simulink model "a11_smlk"  (R2023b)
settings: Solver=ode45  StartTime=0.0  StopTime=3  RelTol=1e-3  EnableMultiTasking=on
values from neighbouring files (symbols this model uses):
  A = [-a-b  0  0 ... (first row only)    [a10_obs_contrls.m]    (also in a11_.m = [ 0   1; a12_.m = [ 0   1; a8_conversao_de_formas.m = [ 0  1; a8_state_space.m = [  0      1)
  alpha = inv((C-D*K)*inv(B*K-A)*B+D)    [a11_.m]    (also in a12_.m; a6_.m = 136.626132179)
  B = [ 1 ... (first row only)    [a10_obs_contrls.m]    (also in a11_.m = [ 0; a12_.m = [ 0; a8_conversao_de_formas.m = [ 0; a8_state_space.m = [ 0)
  C = [0 0 1]    [a10_obs_contrls.m]    (also in a11_.m = [ 1 0 ]; a12_.m = [ 1 0 ]; a3_exercicio.m = (s+2)/(s+1); a8_conversao_de_formas.m = [ 5  3 ])
  D = 0    [a11_.m]    (also in a12_.m; a5_sintonia.m = 1.2; a8_conversao_de_formas.m = 1; a8_state_space.m = [ 0 ])
  K = [ 102 19 ]    [a11_.m]    (also in a12_.m; a3_exercicio.m = 0.0938642036672; a4_exercicio.m = 0.2455; a5_sintonia.m = 23.8830609513)
  r = 45    [a11_.m]    (also in a12_.m)
  x0 = [ 30 ... (first row only)    [a11_.m]    (also in a12_.m; a8_state_space.m = [ 1)
settings Model: Creator=andre.bergmann  LastModifiedBy=LUCAS
settings SolverCC: AlgebraicLoopSolver=TrustRegion
settings DataIOCC: LimitDataPoints=on  SaveFormat=Array  ReturnWorkspaceOutputs=off
settings OptimizationCC: ExpressionDepthLimit=2147483647  LifeSpan=inf
settings DebuggingCC: UnderspecifiedInitializationDetection=Classic  MergeDetectMultiDrivingBlocksExec=none  SolverPrmCheckMsg=warning  UnconnectedInputMsg=warning  UnconnectedOutputMsg=warning  UnconnectedLineMsg=warning  StateNameClashWarn=warning  SFUnexpectedBacktrackingDiag=warning  SFNoUnconditionalDefaultTransitionDiag=warning  SFExecutionAtInitializationDiag=none  ArithmeticOperatorsInVariantConditions=warning
settings HardwareCC: ProdBitPerPointer=32  ProdBitPerSizeT=32  ProdBitPerPtrDiffT=32  ProdLargestAtomicFloat=None  ProdIntDivRoundTo=Undefined  ProdEndianess=Unspecified  ProdWordSize=32  ProdHWDeviceType=32-bit Generic
settings ModelReferenceCC: PropagateSignalLabelsOutOfModel=off
settings SFSimCC: SimUseLocalCustomCode=off  CustomCodeUndefinedFunction=UseInterfaceOnly
settings RTWCC: RTWUseLocalCustomCode=off
settings CodeAppCC: StateflowObjectComments=on
settings GRTTargetCC: TargetLangStandard=C89/C90 (ANSI)
settings ConfigComp: CovMetricSettings=dw  CovSaveCumulativeToWorkspaceVar=on  CovSaveSingleToWorkspaceVar=on  CovExternalEMLEnable=off

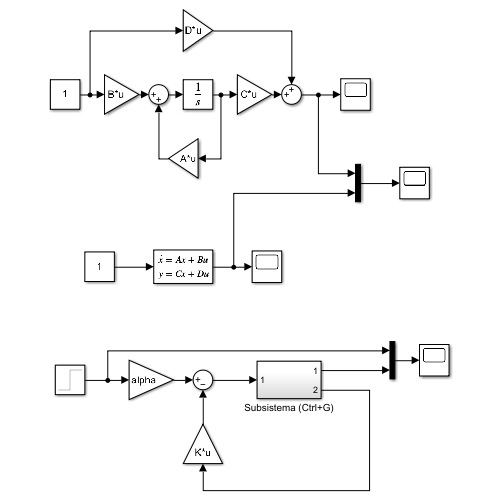
[thumbnail: Simulink's stored preview of the top-level diagram]
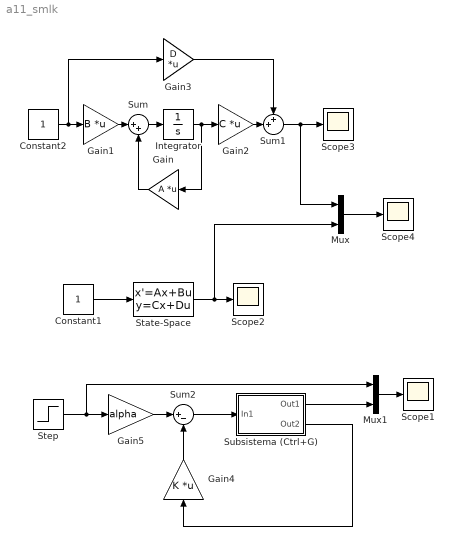
== system a11_smlk ==
  Constant1 : Constant
  Constant2 : Constant
  Gain : Gain  Gain=A  Multiplication=Matrix(K*u)
  Gain1 : Gain  Gain=B  Multiplication=Matrix(K*u)
  Gain2 : Gain  Gain=C  Multiplication=Matrix(K*u)
  Gain3 : Gain  Gain=D  Multiplication=Matrix(K*u)
  Gain4 : Gain  Gain=K  Multiplication=Matrix(K*u)
  Gain5 : Gain  Gain=alpha
  Integrator : Integrator  InitialCondition=x0
  Mux : Mux  Inputs=2
  Mux1 : Mux  Inputs=2
  Scope{1..4} (4 alike) : Scope
  State-Space : StateSpace  A=A  B=B  C=C  D=D  InitialCondition=x0
  Step : Step  After=r  SampleTime=0
  Subsistema (Ctrl+G) : Subsystem
  Sum : Sum  Inputs=|++
  Sum1 : Sum  Inputs=++|
  Sum2 : Sum  Inputs=|+-
  wires:
  Sum2/1 -> Subsistema (Ctrl+G)/1(In1)
  Subsistema (Ctrl+G)/1(Out1) -> Mux1/2
  Subsistema (Ctrl+G)/2(Out2) -> Gain4/1
  Constant1/1 -> State-Space/1
  State-Space/1 -> Mux/2, Scope2/1
  Constant2/1 -> Gain3/1, Gain1/1
  Gain/1 -> Sum/2
  Sum/1 -> Integrator/1
  Sum1/1 -> Mux/1, Scope3/1
  Gain2/1 -> Sum1/2
  Integrator/1 -> Gain2/1, Gain/1
  Gain3/1 -> Sum1/1
  Gain1/1 -> Sum/1
  Mux/1 -> Scope4/1
  Mux1/1 -> Scope1/1
  Gain4/1 -> Sum2/2
  Step/1 -> Mux1/1, Gain5/1
  Gain5/1 -> Sum2/1

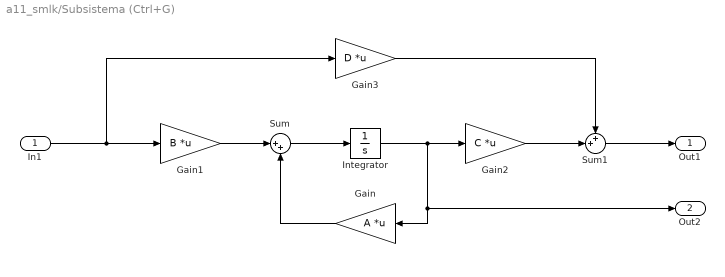
== system a11_smlk/Subsistema (Ctrl+G) ==
  In1 : Inport
  Gain : Gain  Gain=A  Multiplication=Matrix(K*u)
  Gain1 : Gain  Gain=B  Multiplication=Matrix(K*u)
  Gain2 : Gain  Gain=C  Multiplication=Matrix(K*u)
  Gain3 : Gain  Gain=D  Multiplication=Matrix(K*u)
  Integrator : Integrator  InitialCondition=x0
  Sum : Sum  Inputs=|++
  Sum1 : Sum  Inputs=++|
  Out1 : Outport
  Out2 : Outport  Port=2
  wires:
  Gain1/1 -> Sum/1
  Gain2/1 -> Sum1/2
  In1/1 -> Gain3/1, Gain1/1
  Sum1/1 -> Out1/1
  Sum/1 -> Integrator/1
  Gain3/1 -> Sum1/1
  Gain/1 -> Sum/2
  Integrator/1 -> Out2/1, Gain/1, Gain2/1
